simulink model "lab1_model2"  (R2021b)
settings: Solver=VariableStepAuto  StartTime=0.0  StopTime=60  RelTol=1e-3
libraries: cstblocks x4
settings Model: Creator=12288  LastModifiedBy=12288

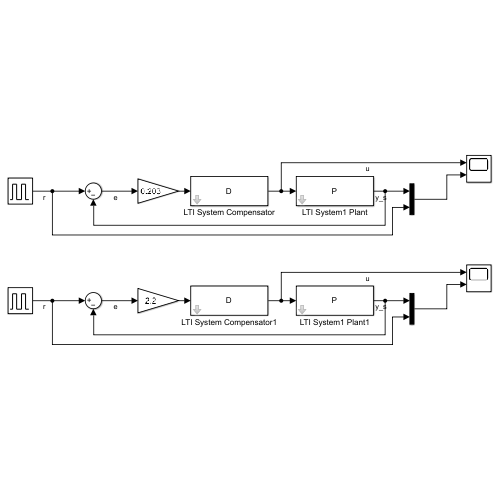
[thumbnail: Simulink's stored preview of the top-level diagram]
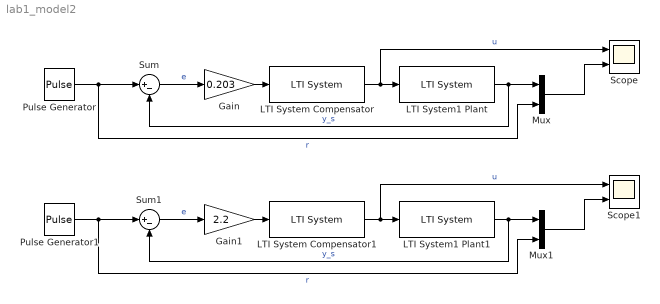
== system lab1_model2 ==
  Gain : Gain  Gain=0.203
  Gain1 : Gain  Gain=2.2
  LTI System Compensator : cstblocks/LTI System  sys=D  IC=[]
  LTI System Compensator1 : cstblocks/LTI System  sys=D  IC=[]
  LTI System1 Plant : cstblocks/LTI System  sys=P  IC=[]
  LTI System1 Plant1 : cstblocks/LTI System  sys=P  IC=[]
  Mux : Mux  Inputs=2
  Mux1 : Mux  Inputs=2
  Pulse Generator : DiscretePulseGenerator  PulseType=Time based  Period=10  PulseWidth=50
  Pulse Generator1 : DiscretePulseGenerator  PulseType=Time based  Period=10  PulseWidth=50
  Scope : Scope  NumInputPorts=2
  Scope1 : Scope  NumInputPorts=2
  Sum : Sum  Inputs=|+-
  Sum1 : Sum  Inputs=|+-
  wires:
  Pulse Generator/1 -> Mux/2, Sum/1  "r"
  Sum/1 -> Gain/1  "e"
  Gain/1 -> LTI System Compensator/1
  LTI System Compensator/1 -> Scope/1, LTI System1 Plant/1  "u"
  LTI System1 Plant/1 -> Sum/2, Mux/1  "y_s"
  Mux/1 -> Scope/2
  Pulse Generator1/1 -> Mux1/2, Sum1/1  "r"
  Sum1/1 -> Gain1/1  "e"
  LTI System1 Plant1/1 -> Sum1/2, Mux1/1  "y_s"
  Gain1/1 -> LTI System Compensator1/1
  Mux1/1 -> Scope1/2
  LTI System Compensator1/1 -> Scope1/1, LTI System1 Plant1/1  "u"
